simulink model "FLCU_Gauging_Test_Harness_WetHeight"  (R2019b)
settings: Solver=FixedStepAuto  StartTime=0.0  StopTime=10  FixedStep=0.02  RelTol=1e-3
settings Model: DataDictionary=FLCU_Gauging.sldd  Creator=aymanouchker  LastModifiedBy=aymanouchker
settings DataIOCC: SignalLoggingName=BusData
settings OptimizationCC: DefaultParameterBehavior=Inlined  UseDivisionForNetSlopeComputation=on  GainParamInheritBuiltInType=on  UseFloatMulNetSlope=on  DefaultUnderspecifiedDataType=single  UseSpecifiedMinMax=on  InlineInvariantSignals=on  EnhancedBackFolding=on  CachingGlobalReferences=on  PassReuseOutputArgsAs=Individual arguments  StateBitsets=on  DataBitsets=on  ZeroExternalMemoryAtStartup=off  ZeroInternalMemoryAtStartup=off  NoFixptDivByZeroProtection=on  EfficientFloat2IntCast=on  LifeSpan=inf  OptimizeBlockOrder=speed  DifferentSizesBufferReuse=on  EfficientTunableParamExpr=on
settings DebuggingCC: SignalInfNanChecking=warning  IntegerOverflowMsg=error  ParameterTunabilityLossMsg=error  UniqueDataStoreMsg=error  AssertControl=DisableAll  StrictBusMsg=ErrorOnBusTreatedAsVector  SFUndirectedBroadcastEventsDiag=error
settings HardwareCC: ProdBitPerInt=16  ProdBitPerPointer=16  ProdBitPerSizeT=16  ProdBitPerPtrDiffT=16  ProdLargestAtomicFloat=None  ProdWordSize=16  ProdLongLongMode=on  ProdHWDeviceType=STMicroelectronics->ST10/Super10
settings SFSimCC: CompileTimeRecursionLimit=0  EnableRuntimeRecursion=off  MATLABDynamicMemAlloc=off
settings RTWCC: SystemTargetFile=ert.tlc  TemplateMakefile=ert_default_tmf  GenerateReport=on  BuildConfiguration=Faster Runs  IncludeHyperlinkInReport=on  LaunchReport=on  GenerateTraceInfo=on  GenerateTraceReport=on  GenerateTraceReportSl=on  GenerateTraceReportSf=on  GenerateTraceReportEml=on
settings CodeAppCC: ForceParamTrailComments=on  IgnoreCustomStorageClasses=off  IgnoreTestpoints=on  OperatorAnnotations=on  SimulinkDataObjDesc=on  SFDataObjDesc=on  MATLABFcnDesc=on  InsertBlockDesc=on  StateflowObjectComments=on  MATLABSourceComments=on  EnableCustomComments=on  ReqsInCode=on
settings ERTTargetCC: TargetLangStandard=C99 (ISO)  UtilityFuncGeneration=Shared location  GenerateSampleERTMain=on  CombineSignalStateStructs=on  SuppressErrorStatus=on  SupportAbsoluteTime=off  MultiInstanceERTCode=on  CodeInterfacePackaging=Reusable function  SupportNonFinite=off  ParenthesesLevel=Maximum  CastingMode=Standards  GenerateSharedConstants=off  InlinedParameterPlacement=NonHierarchical  ERTCustomFileTemplate=example_file_process.tlc  PreserveExpressionOrder=on  PreserveIfCondition=on  EnableSignedLeftShifts=off  EnableSignedRightShifts=off

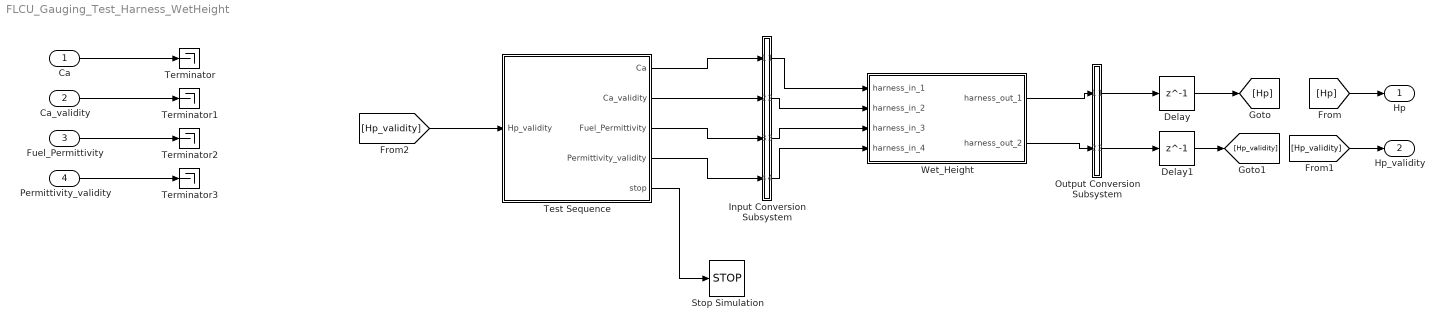
== system FLCU_Gauging_Test_Harness_WetHeight ==
  Ca : Inport  OutDataTypeStr=double  PortDimensions=[1]  SampleTime=[-1, 0]
  Ca_validity : Inport  Port=2  OutDataTypeStr=boolean  PortDimensions=[1]  SampleTime=[-1, 0]
  Fuel_Permittivity : Inport  Port=3  OutDataTypeStr=double  PortDimensions=[1]  SampleTime=[-1, 0]
  Permittivity_validity : Inport  Port=4  OutDataTypeStr=boolean  PortDimensions=[1]  SampleTime=[-1, 0]
  Delay : Delay  DelayLength=1
  Delay1 : Delay  DelayLength=1
  Input Conversion Subsystem : Subsystem  Tag=__SLT_ICS__  Description=|
      | Signal spec.
      | and routing
      settings: AttributesFormatString=%<Description>
  Output Conversion Subsystem : Subsystem  Tag=__SLT_OCS__  Description=|
      | Signal spec.
      | and routing
      settings: AttributesFormatString=%<Description>
  Stop Simulation : Stop
  Terminator{,1..3} (4 alike) : Terminator
  Test Sequence : Test Sequence  TreatAsAtomicUnit=on
  Wet_Height : Subsystem  Tag=__SL_testing_harness_stub_
  Hp : Outport
  Hp_validity : Outport  Port=2
  wires:
  Input Conversion Subsystem/1(Outport_1) -> Wet_Height/1(harness_in_1)
  Input Conversion Subsystem/2(Outport_2) -> Wet_Height/2(harness_in_2)
  Input Conversion Subsystem/3(Outport_3) -> Wet_Height/3(harness_in_3)
  Input Conversion Subsystem/4(Outport_4) -> Wet_Height/4(harness_in_4)
  Wet_Height/1(harness_out_1) -> Output Conversion Subsystem/1(Inport_1)
  Wet_Height/2(harness_out_2) -> Output Conversion Subsystem/2(Inport_2)
  Permittivity_validity/1 -> Terminator3/1
  Ca/1 -> Terminator/1
  Ca_validity/1 -> Terminator1/1
  Fuel_Permittivity/1 -> Terminator2/1
  Test Sequence/5(stop) -> Stop Simulation/1
  Test Sequence/4(Permittivity_validity) -> Input Conversion Subsystem/4(Inport_4)
  Test Sequence/3(Fuel_Permittivity) -> Input Conversion Subsystem/3(Inport_3)
  Test Sequence/2(Ca_validity) -> Input Conversion Subsystem/2(Inport_2)
  Test Sequence/1(Ca) -> Input Conversion Subsystem/1(Inport_1)
  Output Conversion Subsystem/2(Outport_2) -> Delay1/1
  Output Conversion Subsystem/1(Outport_1) -> Delay/1
  Delay/1 -> [Hp]
  Delay1/1 -> [Hp_validity]
  [Hp_validity] -> Hp_validity/1
  [Hp] -> Hp/1
  [Hp_validity] -> Test Sequence/1(Hp_validity)

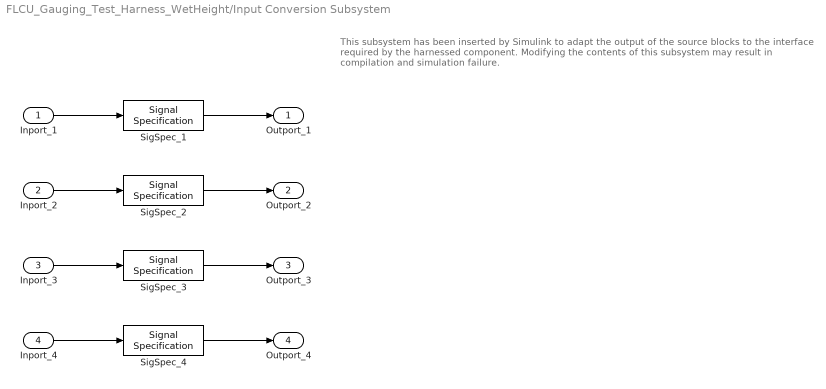
== system FLCU_Gauging_Test_Harness_WetHeight/Input Conversion Subsystem ==
  note: This subsystem has been inserted by Simulink to adapt the output of the source blocks to the interface required by the harnessed component.
      |  Modifying the contents of this subsystem may result in compilation and simulation failure.
  Inport_1 : Inport
  Inport_2 : Inport  Port=2
  Inport_3 : Inport  Port=3
  Inport_4 : Inport  Port=4
  SigSpec_1 : SignalSpecification  OutDataTypeStr=double  Unit=pF  Dimensions=[1]  SampleTime=[-1, 0]
  SigSpec_2 : SignalSpecification  OutDataTypeStr=boolean  Dimensions=[1]  SampleTime=[-1, 0]
  SigSpec_3 : SignalSpecification  OutDataTypeStr=double  Dimensions=[1]  SampleTime=[-1, 0]
  SigSpec_4 : SignalSpecification  OutDataTypeStr=boolean  Dimensions=[1]  SampleTime=[-1, 0]
  Outport_1 : Outport
  Outport_2 : Outport  Port=2
  Outport_3 : Outport  Port=3
  Outport_4 : Outport  Port=4
  wires:
  SigSpec_1/1 -> Outport_1/1
  Inport_1/1 -> SigSpec_1/1
  SigSpec_2/1 -> Outport_2/1
  Inport_2/1 -> SigSpec_2/1
  SigSpec_3/1 -> Outport_3/1
  Inport_3/1 -> SigSpec_3/1
  SigSpec_4/1 -> Outport_4/1
  Inport_4/1 -> SigSpec_4/1

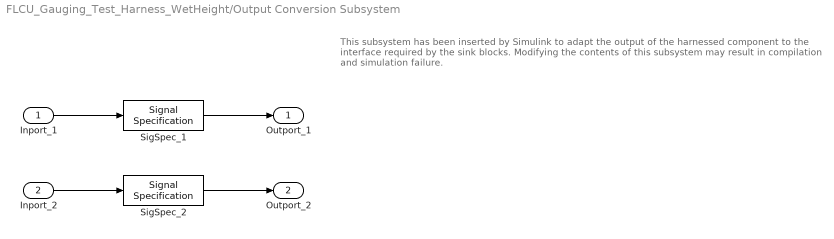
== system FLCU_Gauging_Test_Harness_WetHeight/Output Conversion Subsystem ==
  note: This subsystem has been inserted by Simulink to adapt the output of the harnessed component to the interface required by the sink blocks.
      |  Modifying the contents of this subsystem may result in compilation and simulation failure.
  Inport_1 : Inport
  Inport_2 : Inport  Port=2
  SigSpec_1 : SignalSpecification  OutDataTypeStr=double  Unit=mm  Dimensions=[1]
  SigSpec_2 : SignalSpecification  OutDataTypeStr=boolean  Dimensions=[1]
  Outport_1 : Outport
  Outport_2 : Outport  Port=2
  wires:
  Inport_1/1 -> SigSpec_1/1
  SigSpec_1/1 -> Outport_1/1
  Inport_2/1 -> SigSpec_2/1
  SigSpec_2/1 -> Outport_2/1

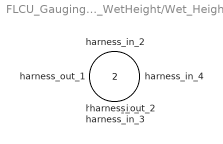
== system FLCU_Gauging_Test_Harness_WetHeight/Wet_Height ==
  harness_in_1 : Inport
  harness_in_2 : Inport  Port=2
  harness_in_3 : Inport  Port=3
  harness_in_4 : Inport  Port=4
  harness_out_1 : Outport
  harness_out_2 : Outport  Port=2

== stateflow chart FLCU_Gauging_Test_Harness_WetHeight/Test Sequence ==
  settings: stateMachineType=SIMPLIFIED_MACHINE
  state Initialization
    Ca=0;
    Ca_validity=true;
    Fuel_Permittivity=0;
    Permittivity_validity=true;
    stop=false;
    count=0;
  state step_1
    Ca=10;
    Ca_validity=true;
    Fuel_Permittivity=2;
    Permittivity_validity=true;
  state step_2
    verify(Hp_validity==true);
  state step_3
    Ca=30000;
    Ca_validity=false;
    Fuel_Permittivity=10;
    Permittivity_validity=false;
  state step_4
    count=count+1;
    verify(Hp_validity==false);
  state step_5
    Ca= 10000;
    Ca_validity=false;
    Fuel_Permittivity=5;
    Permittivity_validity=true;
  state step_6
    Ca=1000;
    Ca_validity=false;
    Fuel_Permittivity=3;
    Permittivity_validity=true;
  state step_8
    Ca= 1000;
    Ca_validity=false;
    Fuel_Permittivity=3;
    Permittivity_validity=false;
  state step_9
    stop=true;
  (default) -> Initialization
  Initialization -> step_1
  step_1 -> step_2
  step_2 -> step_3
  step_3 -> step_4
  (junction 132) -> step_4
  (junction 154) -> (junction 132)
  step_4 -> (junction 150) [order 4] : [
      | count==4
      | ]
  (junction 150) -> (junction 148)
  step_4 -> (junction 159) [order 2] : [
      | count==2
      | ]
  (junction 159) -> (junction 140)
  step_4 -> (junction 161) [order 3] : [
      | count==3
      | ]
  (junction 161) -> (junction 144)
  step_4 -> step_5 [order 1] : [
      | count==1
      | ]
  step_5 -> step_4
  step_6 -> (junction 154)
  (junction 140) -> step_6
  (junction 134) -> (junction 154)
  step_8 -> (junction 134)
  (junction 144) -> step_8
  (junction 148) -> step_9
  data: Hp_validity input; Ca output; Ca_validity output; Fuel_Permittivity output; Permittivity_validity output; stop output; count local
